simulink model "PI_lead"  (R2023b)
settings: Solver=ode8  StartTime=0.0  StopTime=20  FixedStep=0.005  RelTol=1e-3
values from neighbouring files (symbols this model uses):
  K = p/z    [lead_vs_leadlag.m]    (also in setup_lead_controller.m)
  p = bodeoptions    [PID_lead_linmod.m]    (also in lead_vs_leadlag.m = 1/(alpha*T); setup_lead_controller.m = 1/(alpha*T))
  z = 1/T    [lead_vs_leadlag.m]    (also in setup_lead_controller.m)
settings Model: Creator=suvo  LastModifiedBy=suvo
settings SolverCC: AlgebraicLoopSolver=TrustRegion
settings DataIOCC: ReturnWorkspaceOutputs=off
settings DebuggingCC: UnconnectedInputMsg=warning  UnconnectedOutputMsg=warning  UnconnectedLineMsg=warning
settings ModelReferenceCC: EnableRefExpFcnMdlSchedulingChecks=on

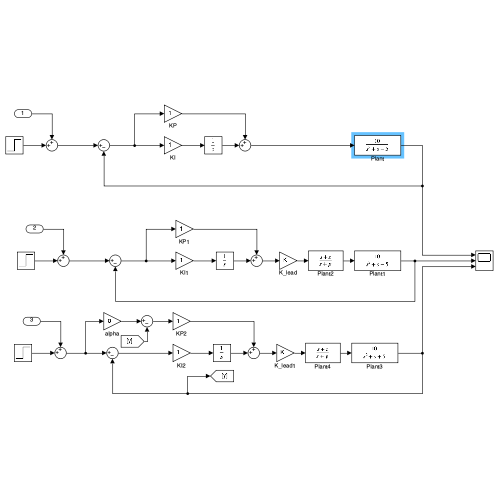
[thumbnail: Simulink's stored preview of the top-level diagram]
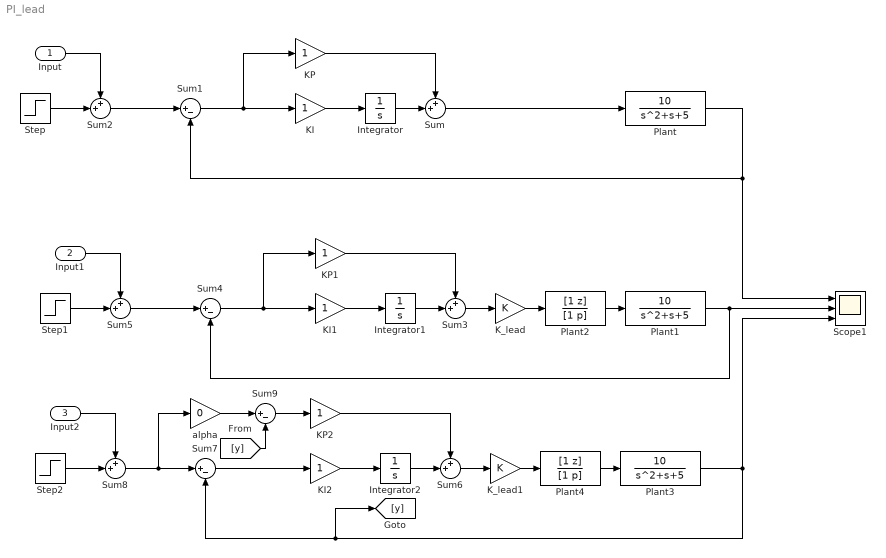
== system PI_lead ==
  Input : Inport
  Input1 : Inport  Port=2
  Input2 : Inport  Port=3
  Integrator : Integrator
  Integrator1 : Integrator
  Integrator2 : Integrator
  KI : Gain
  KI1 : Gain
  KI2 : Gain
  KP : Gain
  KP1 : Gain
  KP2 : Gain
  K_lead : Gain  Gain=K
  K_lead1 : Gain  Gain=K
  Plant : TransferFcn  Numerator=10  Denominator=[1 1 5]
  Plant1 : TransferFcn  Numerator=10  Denominator=[1 1 5]
  Plant2 : TransferFcn  Numerator=[1 z]  Denominator=[1 p]
  Plant3 : TransferFcn  Numerator=10  Denominator=[1 1 5]
  Plant4 : TransferFcn  Numerator=[1 z]  Denominator=[1 p]
  Scope1 : Scope  NumInputPorts=3
  Step : Step  SampleTime=0
  Step1 : Step  SampleTime=0
  Step2 : Step  SampleTime=0
  Sum{,2..3,5..6,8} (6 alike) : Sum  Inputs=++|
  Sum{1,4,7,9} (4 alike) : Sum  Inputs=|+-
  alpha : Gain  Gain=0
  wires:
  KI/1 -> Integrator/1
  Sum1/1 -> KP/1, KI/1
  KP/1 -> Sum/1
  Integrator/1 -> Sum/2
  Sum/1 -> Plant/1
  Plant/1 -> Sum1/2, Scope1/1
  Step/1 -> Sum2/2
  Input/1 -> Sum2/1
  Sum2/1 -> Sum1/1
  Plant1/1 -> Sum4/2, Scope1/2
  Sum4/1 -> KP1/1, KI1/1
  KP1/1 -> Sum3/1
  KI1/1 -> Integrator1/1
  Integrator1/1 -> Sum3/2
  Plant2/1 -> Plant1/1
  Sum3/1 -> K_lead/1
  Input1/1 -> Sum5/1
  Sum5/1 -> Sum4/1
  Step1/1 -> Sum5/2
  K_lead/1 -> Plant2/1
  Input2/1 -> Sum8/1
  Sum6/1 -> K_lead1/1
  Step2/1 -> Sum8/2
  Plant4/1 -> Plant3/1
  Plant3/1 -> Scope1/3, [y], Sum7/2
  Integrator2/1 -> Sum6/2
  KI2/1 -> Integrator2/1
  Sum8/1 -> alpha/1, Sum7/1
  KP2/1 -> Sum6/1
  Sum7/1 -> KI2/1
  K_lead1/1 -> Plant4/1
  Sum9/1 -> KP2/1
  [y] -> Sum9/2
  alpha/1 -> Sum9/1
